simulink model "sfcndemo_sfun_rtwdwork"  (Simulink 7.6)
settings: Solver=FixedStepDiscrete  StartTime=0.0  StopTime=10.0  FixedStep=1  RelTol=1e-3
Description:
  | DWork S-function example, including Real-Time Workshop considerations
settings Model: Creator=The MathWorks Inc.  ExtModeAutoUpdateStatusClock=off
settings OptimizationCC: BooleanDataType=off  InlineParams=on  ZeroExternalMemoryAtStartup=off  ZeroInternalMemoryAtStartup=off  OptimizeModelRefInitCode=on  LifeSpan=1
settings DebuggingCC: SaveWithParameterizedLinksMsg=none  SignalResolutionControl=TryResolveAllWithWarning  SolverPrmCheckMsg=none  MultiTaskDSMMsg=warning  MultiTaskCondExecSysMsg=none
settings HardwareCC: TargetUnknown=on
settings RTWCC: SystemTargetFile=ert.tlc  GenCodeOnly=on  TemplateMakefile=ert_default_tmf  ProcessScript=ert_make_rtw_hook  IncludeERTFirstTime=on
settings CodeAppCC: IgnoreCustomStorageClasses=off  CustomSymbolStrFcn=$F$N$M
settings ERTTargetCC: TargetFcnLib=ansi_tfl_tmw.mat  MultiwordLength=2048  GenerateSampleERTMain=on  InlinedParameterPlacement=NonHierarchical  ERTCustomFileTemplate=example_file_process.tlc  ConvertIfToSwitch=off

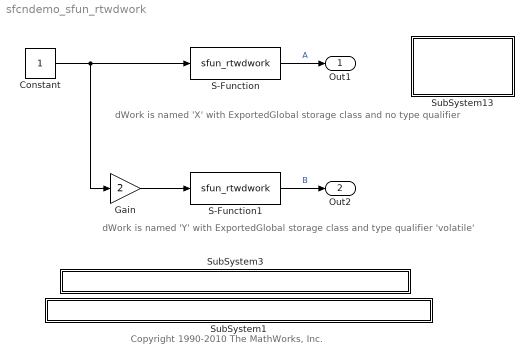
== system sfcndemo_sfun_rtwdwork ==
  note: dWork is named 'X' with ExportedGlobal
      | storage class and no type qualifier
  note: dWork is named 'Y' with ExportedGlobal
      | storage class and type qualifier 'volatile'
  note: Copyright 1990-2010 The MathWorks, Inc.
  Constant : Constant
  Gain : Gain  Gain=2  OutDataTypeStr=Inherit: Same as input  ParamDataTypeStr=Inherit: Same as input
  S-Function : S-Function  FunctionName=sfun_rtwdwork  Parameters=id,sc,tq  EnableBusSupport=off  mask{id='X', sc=ExportedGlobal, tq=''}
      mask prompts: id "RTW Identifier"; sc "RTW Storage Class"; tq "RTW Type Qualifier"
      mask StyleString: edit,popup(Auto|ExportedGlobal|ImportedExtern|ImportedExternPointer),edit
  S-Function1 : S-Function  FunctionName=sfun_rtwdwork  Parameters=id,sc,tq  EnableBusSupport=off  mask{id='Y', sc=ExportedGlobal, tq='volatile'}
      mask prompts: id "RTW Identifier"; sc "RTW Storage Class"; tq "RTW Type Qualifier"
      mask StyleString: edit,popup(Auto|ExportedGlobal|ImportedExtern|ImportedExternPointer),edit
  SubSystem1 : Subsystem  mask{filename=sfun_rtwdwork.tlc}
      mask init:
      | x=sfundemo_maskdisp;
      settings: AttributesFormatString=\n  OpenFcn=sfundemo_openfcn
      mask Display: disp(x);
  SubSystem13 : Subsystem
      settings: OpenFcn=rtwdwork_inspect('sfcndemo_sfun_rtwdwork.c');
      mask Display: disp('Generate and\ninspect code')
  SubSystem3 : Subsystem  mask{filename=sfun_rtwdwork.c}
      mask init:
      | x=sfundemo_maskdisp;
      settings: AttributesFormatString=\n  OpenFcn=sfundemo_openfcn
      mask Display: disp(x);
  Out1 : Outport
  Out2 : Outport  Port=2
  wires:
  Constant/1 -> S-Function/1, Gain/1
  S-Function/1 -> Out1/1  "A"
  S-Function1/1 -> Out2/1  "B"
  Gain/1 -> S-Function1/1

== system sfcndemo_sfun_rtwdwork/SubSystem1 ==

== system sfcndemo_sfun_rtwdwork/SubSystem13 ==

== system sfcndemo_sfun_rtwdwork/SubSystem3 ==
